simulink model "SystemLQR"  (R2023a)
settings: Solver=VariableStepAuto  StartTime=0.0  StopTime=10.0  MaxStep=0.01  RelTol=1e-3  AbsTol=1e-3  EnableMultiTasking=on
undefined symbols (not defined in the file): DemoControllers
settings Model: Creator=KozlovM  LastModifiedBy=diontep
settings SolverCC: AutoScaleAbsTol=off  AlgebraicLoopSolver=TrustRegion  MaxZcPerStep=1
settings DataIOCC: LimitDataPoints=on  MaxDataPoints=10000
settings OptimizationCC: ReuseModelBlockBuffer=off  LifeSpan=inf
settings DebuggingCC: UnconnectedInputMsg=warning  UnconnectedOutputMsg=warning  UnconnectedLineMsg=warning  AllowSymbolicDim=off  SubsystemReferenceDiagnosticForUnitTest=warning  SFUnexpectedBacktrackingDiag=warning  SFNoUnconditionalDefaultTransitionDiag=warning  SFExecutionAtInitializationDiag=none  ArithmeticOperatorsInVariantConditions=warning
settings ModelReferenceCC: EnableRefExpFcnMdlSchedulingChecks=on
settings SFSimCC: SimUseLocalCustomCode=off  CustomCodeUndefinedFunction=UseInterfaceOnly
settings RTWCC: RTWUseLocalCustomCode=off  DLArmComputeVersion=19.05
settings CodeAppCC: StateflowObjectComments=on
settings GRTTargetCC: TargetLangStandard=C89/C90 (ANSI)
settings ConfigComp: CovMetricSettings=dw  CovSaveCumulativeToWorkspaceVar=on  CovSaveSingleToWorkspaceVar=on  CovExternalEMLEnable=off  CovSFcnEnable=off
settings SimscapeCC: SimscapeLogType=all  SimscapeLogSimulationStatistics=on  SimscapeLogDataHistory=10000

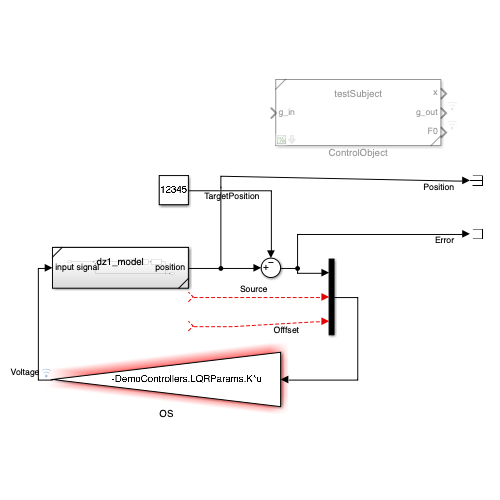
[thumbnail: Simulink's stored preview of the top-level diagram]
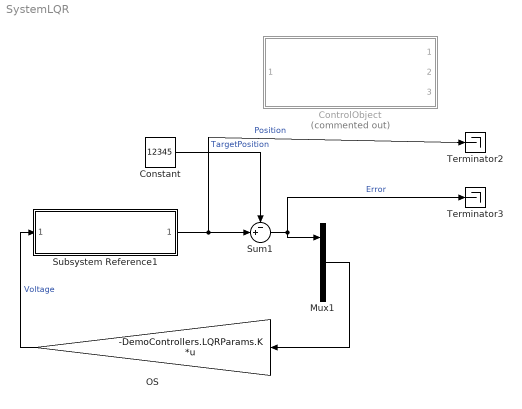
== system SystemLQR ==
  Constant : Constant  Value=12345
  ControlObject : Subsystem  Commented=on  ReferencedSubsystem=testSubject
  Mux1 : Mux  Inputs=3
  OS : Gain  Gain=-DemoControllers.LQRParams.K  Multiplication=Matrix(K*u)
  Subsystem Reference1 : Subsystem  ReferencedSubsystem=dz1_model
  Sum1 : Sum  Inputs=-+|
  Terminator2 : Terminator
  Terminator3 : Terminator
  wires:
  Subsystem Reference1/1 -> Terminator2/1, Sum1/2  "Position"
  Constant/1 -> Sum1/1  "TargetPosition"
  Mux1/1 -> OS/1
  ? -> Mux1/2  "Source"
  ? -> Mux1/3  "Offfset"
  Sum1/1 -> Terminator3/1, Mux1/1  "Error"
  OS/1 -> Subsystem Reference1/1  "Voltage"
